simulink model "untitled"  (R2018a)
settings: Solver=VariableStepAuto  StartTime=0.0  StopTime=40  RelTol=1e-3
settings Model: Creator=bssho  LastModifiedBy=bssho

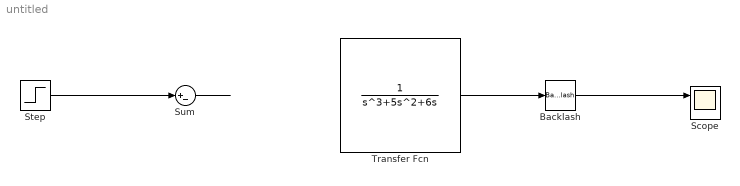
== system untitled ==
  Backlash : Backlash
  Scope : Scope  NumInputPorts=2
  Step : Step  SampleTime=0
  Sum : Sum  Inputs=|+-
  Transfer Fcn : TransferFcn  Denominator=[1 5 6 0]
  wires:
  ? -> Transfer Fcn/1
  Step/1 -> Sum/1
  Sum/1 -> ?
  Backlash/1 -> Scope/1
  Transfer Fcn/1 -> Backlash/1
